simulink model "MASK_demodulation"  (R2016a)
settings: Solver=VariableStepAuto  StartTime=0.0  StopTime=9/Fd  RelTol=1e-3
values from neighbouring files (symbols this model uses):
  Fc = 2e6    (= 2000000)    [MASK.m]
  Fd = 200e3    (= 200000)    [MASK.m]
  Fs = 50e6    (= 50000000)    [MASK.m]
libraries: commchan3 x1, dsparch4 x1, simulink x1
settings Model: Creator=ZM  LastModifiedBy=ZM

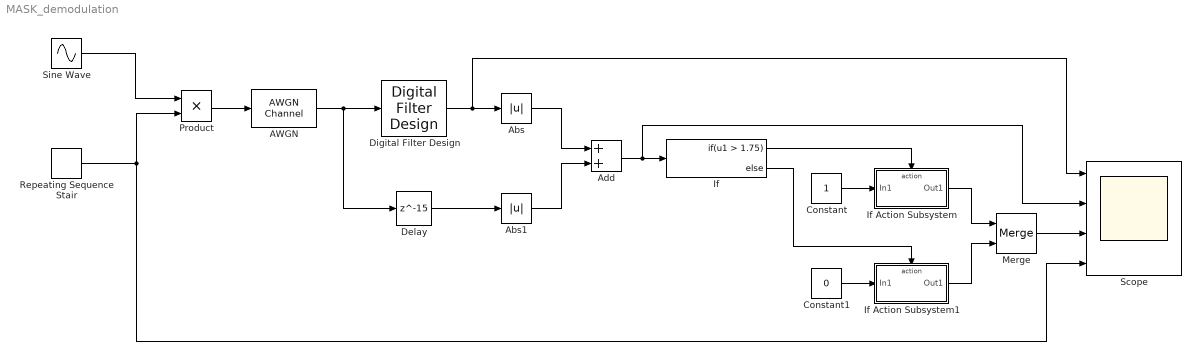
== system MASK_demodulation ==
  "AWGN " : commchan3/AWGN Channel  InputProcessing=Columns as channels (frame based)  seed=67  noiseMode="Signal to noise ratio  (SNR)"  EbNodB=100  EsNodB=10  SNRdB=20  bitsPerSym=1  Ps=1  Tsym=1  variance=1
  Abs : Abs
  Abs1 : Abs
  Add : Sum
  Constant : Constant
  Constant1 : Constant  Value=0
  Delay : Delay  DelayLength=15  InitialCondition=0
  Digital Filter Design : dsparch4/Digital Filter Design  mwdsp_browser_bugfix_var=off
  If : If  IfExpression=u1 > 1.75
  If Action Subsystem : Subsystem  TreatAsAtomicUnit=on
  If Action Subsystem1 : Subsystem  TreatAsAtomicUnit=on
  Merge : Merge  InitialOutput=[0]
  Product : Product
  Repeating Sequence Stair : simulink/Sources/Repeating Sequence Stair  OutValues=[2 2 1 2 1 1 1 2 2].'  tsamp=1/Fd  OutMin=[]  OutMax=[]  OutDataTypeStr=double  OutputDataTypeScalingMode=double  OutDataType=fixdt(0,8)  ConRadixGroup=Best Precision: Vector-wise  OutScaling=2^-12
  Scope : Scope  NumInputPorts=4
  Sine Wave : Sin  Frequency=2*pi*Fc  SampleTime=1/Fs
  wires:
  Digital Filter Design/1 -> Scope/1, Abs/1
  Delay/1 -> Abs1/1
  Abs/1 -> Add/1
  Abs1/1 -> Add/2
  Sine Wave/1 -> Product/1
  Repeating Sequence Stair/1 -> Scope/4, Product/2
  Add/1 -> Scope/2, If/1
  If/1 -> If Action Subsystem/Action
  Constant/1 -> If Action Subsystem/1(In1)
  If/2 -> If Action Subsystem1/Action
  Constant1/1 -> If Action Subsystem1/1(In1)
  If Action Subsystem/1(Out1) -> Merge/1
  If Action Subsystem1/1(Out1) -> Merge/2
  Merge/1 -> Scope/3
  Product/1 -> "AWGN "/1
  "AWGN "/1 -> Digital Filter Design/1, Delay/1

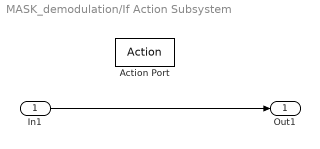
== system MASK_demodulation/If Action Subsystem ==
  In1 : Inport
  Action Port : ActionPort  ActionType=then
  Out1 : Outport
  wires:
  In1/1 -> Out1/1

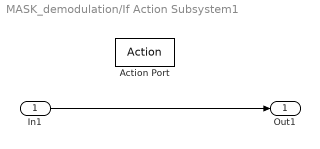
== system MASK_demodulation/If Action Subsystem1 ==
  In1 : Inport
  Action Port : ActionPort  ActionType=else
  Out1 : Outport
  wires:
  In1/1 -> Out1/1
